simulink model "shoot"  (R2017b)
settings: Solver=VariableStepAuto  StartTime=0.0  StopTime=10.0  RelTol=1e-3
settings Model: Creator=ghleila  LastModifiedBy=ghleila

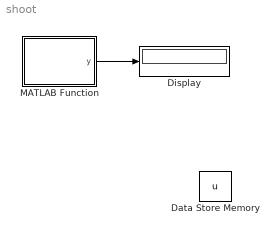
== system shoot ==
  Data Store Memory : DataStoreMemory  DataStoreName=u  InitialValue=5  ShowAdditionalParam=off  OutDataTypeStr=double
  Display : Display
  MATLAB Function : MATLAB Function  TreatAsAtomicUnit=on
  wires:
  MATLAB Function/1(y) -> Display/1

== matlab function shoot/MATLAB Function ==
  data: y output
function y = fcn


global U;
U = U+1;
y = U;
